simulink model "UAVLinCL_SAT"  (R2023a)
settings: Solver=ode45  StartTime=0.0  StopTime=5  RelTol=1e-6  EnableMultiTasking=on
values from neighbouring files (symbols this model uses):
  A = [-0.5572,-0.7814;0.7814,0]    [Calculos02_Vnoladetrim.m]
  B = [1,-1;0,2]    [Calculos02_Vnoladetrim.m]
  C = [1.9691,6.4493]    [Calculos02_Vnoladetrim.m]
  K = Klqr    [Calculos00_OriginalIgnacio.m]    (also in PI_4_OBSOLETE_TestingPredictedController.m = state2k(state); PI_5_PIofVariousPredictedController.m = reshape(DATA(index,3:12), 2, 5); PI_6_Tracker_bigGuy.m = zeros(2,5); PI_9_playground_state2k.m = state2k(state))
  x0 = [-1 0 -0.5 -0.5 0]    [BackUp_Simulation_002.mat]    (also in Calculos00_OriginalIgnacio.m = [0,deltaAoA,0,0,0]; Calculos02_Vnoladetrim.m = [1, 0, 0, 0, 0]; GenerateDataset_v0.m = [-1,0,0,0,0]'; PI_0_OnlyOneController_V20.m = [-1,0,0,0,0]')
undefined symbols (not defined in the file or in its folder): Utrim, Xtrim
settings Model: Creator=Ignacio  LastModifiedBy=ignac
settings SolverCC: AlgebraicLoopSolver=TrustRegion
settings DataIOCC: ExternalInput=[0 0.369809473744665 -0.0760167506859634 0.299999999999976]  InitialState=[]  LimitDataPoints=on  SaveFormat=Array  SignalLoggingSaveFormat=ModelDataLogs  ReturnWorkspaceOutputs=off
settings OptimizationCC: DefaultParameterBehavior=Inlined  BufferReuse=off  ExpressionDepthLimit=2147483647  LifeSpan=inf
settings DebuggingCC: UnderspecifiedInitializationDetection=Classic  MergeDetectMultiDrivingBlocksExec=none  FcnCallInpInsideContextMsg=warning  UnconnectedInputMsg=warning  UnconnectedOutputMsg=warning  UnconnectedLineMsg=warning  StateNameClashWarn=warning  InitInArrayFormatMsg=none  SFUnexpectedBacktrackingDiag=warning  SFNoUnconditionalDefaultTransitionDiag=warning  SFExecutionAtInitializationDiag=none  ArithmeticOperatorsInVariantConditions=warning
settings HardwareCC: ProdBitPerPointer=32  ProdBitPerSizeT=32  ProdBitPerPtrDiffT=32  ProdLargestAtomicFloat=None  ProdIntDivRoundTo=Undefined  ProdEndianess=Unspecified  ProdWordSize=32  ProdHWDeviceType=32-bit Generic
settings ModelReferenceCC: EnableRefExpFcnMdlSchedulingChecks=on  PropagateSignalLabelsOutOfModel=off
settings SFSimCC: SimUseLocalCustomCode=off  CustomCodeUndefinedFunction=UseInterfaceOnly
settings RTWCC: RTWUseLocalCustomCode=off
settings CodeAppCC: StateflowObjectComments=on
settings GRTTargetCC: TargetLangStandard=C89/C90 (ANSI)
settings ConfigComp: CovMetricSettings=dw  CovSaveCumulativeToWorkspaceVar=on  CovSaveSingleToWorkspaceVar=on  CovExternalEMLEnable=off

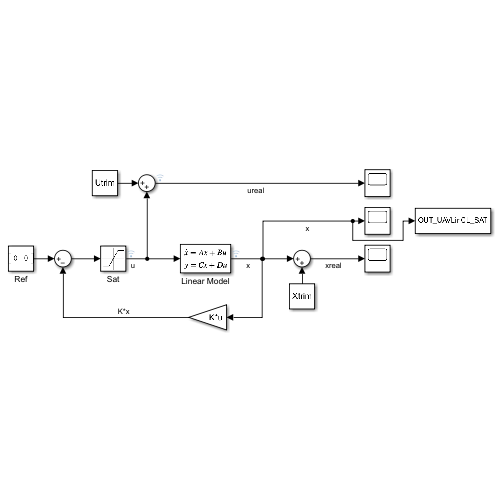
[thumbnail: Simulink's stored preview of the top-level diagram]
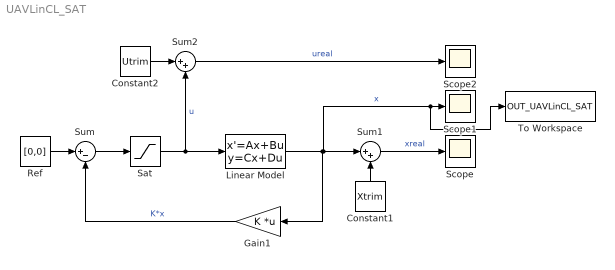
== system UAVLinCL_SAT ==
  Constant1 : Constant  Value=Xtrim
  Constant2 : Constant  Value=Utrim
  Gain1 : Gain  Gain=K  Multiplication=Matrix(K*u)
  Linear Model : StateSpace  A=A  B=B  C=C  D=zeros(5,2)  InitialCondition=x0
  Ref : Constant  Value=[0,0]
  Sat : Saturate  UpperLimit=[1; 0.5] - Utrim  LowerLimit=[0; -0.5] - Utrim
  Scope : Scope
  Scope1 : Scope
  Scope2 : Scope
  Sum : Sum  Inputs=|+-
  Sum1 : Sum  Inputs=|++
  Sum2 : Sum  Inputs=|++
  To Workspace : ToWorkspace  VariableName=OUT_UAVLinCL_SAT  SaveFormat=Timeseries  SampleTime=-1
  wires:
  Linear Model/1 -> To Workspace/1, Scope1/1, Sum1/1, Gain1/1  "x"
  Gain1/1 -> Sum/2  "K*x"
  Ref/1 -> Sum/1
  Sum/1 -> Sat/1
  Constant1/1 -> Sum1/2
  Sum1/1 -> Scope/1  "xreal"
  Sat/1 -> Linear Model/1, Sum2/2  "u"
  Constant2/1 -> Sum2/1
  Sum2/1 -> Scope2/1  "ureal"
